simulink model "P702_NI_SoftECU"  (R2019a)
settings: Solver=ode1  StartTime=0.0  StopTime=Inf  FixedStep=0.001  RelTol=1e-3  EnableMultiTasking=on
PreLoadFcn:
  | run '.\VeriStand_BlockSet\NIVeriStandAddPaths.m'
undefined symbols (not defined in the file or in its folder): magnitude
libraries: simulink x83, simulink_extras x1
(part 2 of 76)

== system P702_NI_SoftECU/Input/GWM-SCCM//PDB//RCM//GSM ==
  Bus Creator : BusCreator  Inputs=5
  GMW_Extra_Disable : S-Function  Priority=1  FunctionName=NIVeriStandIO  Parameters=width dtype portnum stime stype btype  SFunctionDeploymentMode=off  EnableBusSupport=off  mask(NI VeriStand Inport){portnum=1, width=-1, stime=-1, dtype=auto, stype=auto, btype=1}
      mask prompts: portnum "Port number:"; width "Port dimensions (-1 for dynamically sized):"; stime "Sample time (-1 for inherited):"; dtype "Data type:"; stype "Signal type:"; btype "Block type:"
      mask help: Use this inport on any level of nested subsystems to allow NI VeriStand software to map signals to it.
      mask init:
      | NIVeriStandIO_init;
      settings: CopyFcn=NIVeriStand_MDL_functions('', 'IO_copy');  DeleteFcn=NIVeriStand_MDL_functions('', 'IO_delete');  MoveFcn=set_param(gcb, 'Mask', 'on');
      mask Callback portnum: NIVeriStand_MDL_functions('', 'IO_setportnum');
      mask TypeOptions dtype: auto | double | single | int8 | uint8 | int16 | uint16 | int32 | uint32 | boolean
      mask Callback dtype: NIVeriStand_MDL_functions('', 'IO_booleansignal');
      mask TypeOptions stype: auto | real | complex
      mask Display:
      | patch([-x x], [-y y], [.90980 .81960 .32156]);
      | plot([xrad -x x xrad], [yrad -y y yrad]);
      | fprintf('NI In%d', portnum);
  GSM : Subsystem  TreatAsAtomicUnit=on
  GSM_Disable : S-Function  Priority=2  FunctionName=NIVeriStandIO  Parameters=width dtype portnum stime stype btype  SFunctionDeploymentMode=off  EnableBusSupport=off  mask(NI VeriStand Inport){portnum=2, width=-1, stime=-1, dtype=auto, stype=auto, btype=1}
      mask prompts: portnum "Port number:"; width "Port dimensions (-1 for dynamically sized):"; stime "Sample time (-1 for inherited):"; dtype "Data type:"; stype "Signal type:"; btype "Block type:"
      mask help: Use this inport on any level of nested subsystems to allow NI VeriStand software to map signals to it.
      mask init:
      | NIVeriStandIO_init;
      settings: CopyFcn=NIVeriStand_MDL_functions('', 'IO_copy');  DeleteFcn=NIVeriStand_MDL_functions('', 'IO_delete');  MoveFcn=set_param(gcb, 'Mask', 'on');
      mask Callback portnum: NIVeriStand_MDL_functions('', 'IO_setportnum');
      mask TypeOptions dtype: auto | double | single | int8 | uint8 | int16 | uint16 | int32 | uint32 | boolean
      mask Callback dtype: NIVeriStand_MDL_functions('', 'IO_booleansignal');
      mask TypeOptions stype: auto | real | complex
      mask Display:
      | patch([-x x], [-y y], [.90980 .81960 .32156]);
      | plot([xrad -x x xrad], [yrad -y y yrad]);
      | fprintf('NI In%d', portnum);
  Other_GWMTx : Subsystem  TreatAsAtomicUnit=on
  RCM : Subsystem  TreatAsAtomicUnit=on
  RCM_Disable : S-Function  Priority=3  FunctionName=NIVeriStandIO  Parameters=width dtype portnum stime stype btype  SFunctionDeploymentMode=off  EnableBusSupport=off  mask(NI VeriStand Inport){portnum=3, width=-1, stime=-1, dtype=auto, stype=auto, btype=1}
      mask prompts: portnum "Port number:"; width "Port dimensions (-1 for dynamically sized):"; stime "Sample time (-1 for inherited):"; dtype "Data type:"; stype "Signal type:"; btype "Block type:"
      mask help: Use this inport on any level of nested subsystems to allow NI VeriStand software to map signals to it.
      mask init:
      | NIVeriStandIO_init;
      settings: CopyFcn=NIVeriStand_MDL_functions('', 'IO_copy');  DeleteFcn=NIVeriStand_MDL_functions('', 'IO_delete');  MoveFcn=set_param(gcb, 'Mask', 'on');
      mask Callback portnum: NIVeriStand_MDL_functions('', 'IO_setportnum');
      mask TypeOptions dtype: auto | double | single | int8 | uint8 | int16 | uint16 | int32 | uint32 | boolean
      mask Callback dtype: NIVeriStand_MDL_functions('', 'IO_booleansignal');
      mask TypeOptions stype: auto | real | complex
      mask Display:
      | patch([-x x], [-y y], [.90980 .81960 .32156]);
      | plot([xrad -x x xrad], [yrad -y y yrad]);
      | fprintf('NI In%d', portnum);
  SCCM : Subsystem  TreatAsAtomicUnit=on
  SCCM_Disable : S-Function  Priority=4  FunctionName=NIVeriStandIO  Parameters=width dtype portnum stime stype btype  SFunctionDeploymentMode=off  EnableBusSupport=off  mask(NI VeriStand Inport){portnum=4, width=-1, stime=-1, dtype=auto, stype=auto, btype=1}
      mask prompts: portnum "Port number:"; width "Port dimensions (-1 for dynamically sized):"; stime "Sample time (-1 for inherited):"; dtype "Data type:"; stype "Signal type:"; btype "Block type:"
      mask help: Use this inport on any level of nested subsystems to allow NI VeriStand software to map signals to it.
      mask init:
      | NIVeriStandIO_init;
      settings: CopyFcn=NIVeriStand_MDL_functions('', 'IO_copy');  DeleteFcn=NIVeriStand_MDL_functions('', 'IO_delete');  MoveFcn=set_param(gcb, 'Mask', 'on');
      mask Callback portnum: NIVeriStand_MDL_functions('', 'IO_setportnum');
      mask TypeOptions dtype: auto | double | single | int8 | uint8 | int16 | uint16 | int32 | uint32 | boolean
      mask Callback dtype: NIVeriStand_MDL_functions('', 'IO_booleansignal');
      mask TypeOptions stype: auto | real | complex
      mask Display:
      | patch([-x x], [-y y], [.90980 .81960 .32156]);
      | plot([xrad -x x xrad], [yrad -y y yrad]);
      | fprintf('NI In%d', portnum);
  Tester/AutoSar : Subsystem  TreatAsAtomicUnit=on
  Tstr/AutoSar_Disable : S-Function  Priority=5  FunctionName=NIVeriStandIO  Parameters=width dtype portnum stime stype btype  SFunctionDeploymentMode=off  EnableBusSupport=off  mask(NI VeriStand Inport){portnum=5, width=-1, stime=-1, dtype=auto, stype=auto, btype=1}
      mask prompts: portnum "Port number:"; width "Port dimensions (-1 for dynamically sized):"; stime "Sample time (-1 for inherited):"; dtype "Data type:"; stype "Signal type:"; btype "Block type:"
      mask help: Use this inport on any level of nested subsystems to allow NI VeriStand software to map signals to it.
      mask init:
      | NIVeriStandIO_init;
      settings: CopyFcn=NIVeriStand_MDL_functions('', 'IO_copy');  DeleteFcn=NIVeriStand_MDL_functions('', 'IO_delete');  MoveFcn=set_param(gcb, 'Mask', 'on');
      mask Callback portnum: NIVeriStand_MDL_functions('', 'IO_setportnum');
      mask TypeOptions dtype: auto | double | single | int8 | uint8 | int16 | uint16 | int32 | uint32 | boolean
      mask Callback dtype: NIVeriStand_MDL_functions('', 'IO_booleansignal');
      mask TypeOptions stype: auto | real | complex
      mask Display:
      | patch([-x x], [-y y], [.90980 .81960 .32156]);
      | plot([xrad -x x xrad], [yrad -y y yrad]);
      | fprintf('NI In%d', portnum);
  GWM_FD1 : Outport
  wires:
  Bus Creator/1 -> GWM_FD1/1
  Other_GWMTx/1(Other_GWMTx) -> Bus Creator/1  "Other_GWMTx"
  RCM/1(RCM_Signals) -> Bus Creator/2  "RCM"
  SCCM/1(SCCM_Signals) -> Bus Creator/3  "SCCM"
  GSM/1(GSM_Signals) -> Bus Creator/4  "GSM"
  GMW_Extra_Disable/1 -> Other_GWMTx/Enable
  RCM_Disable/1 -> RCM/Enable
  SCCM_Disable/1 -> SCCM/Enable
  GSM_Disable/1 -> GSM/Enable
  Tstr/AutoSar_Disable/1 -> Tester/AutoSar/Enable
  Tester/AutoSar/1(Tester/AutoSar) -> Bus Creator/5  "Tester/AutoSar"

== system P702_NI_SoftECU/Input/PSCM ==
  Enable : EnablePort
  Bus_Msg : BusCreator  Inputs=6
  EPAS_INFO_0x82 : Subsystem
  Lane_Assist_Data3_FD1_0x3CC : Subsystem
  PSCM_AutoSar_NetwrkMgmt_0x5B5 : Subsystem
  SteeringPinion_Data_0x7E : Subsystem
  TesterPhysicalResPSCM_0x738 : Subsystem
  TrailerAid_Data2_0x417 : Subsystem
  PSCM : Outport
  wires:
  Bus_Msg/1 -> PSCM/1  "PSCM"
  SteeringPinion_Data_0x7E/1(SteeringPinion_Data_0x7E) -> Bus_Msg/1  "SteeringPinion_Data_0x7E"
  EPAS_INFO_0x82/1(EPAS_INFO_0x82) -> Bus_Msg/2  "EPAS_INFO_0x82"
  Lane_Assist_Data3_FD1_0x3CC/1(Lane_Assist_Data3_FD1_0x3CC) -> Bus_Msg/3  "Lane_Assist_Data3_FD1_0x3CC"
  TrailerAid_Data2_0x417/1(TrailerAid_Data2_0x417) -> Bus_Msg/4  "TrailerAid_Data2_0x417"
  PSCM_AutoSar_NetwrkMgmt_0x5B5/1(PSCM_AutoSar_NetwrkMgmt_0x5B5) -> Bus_Msg/5  "PSCM_AutoSar_NetwrkMgmt_0x5B5"
  TesterPhysicalResPSCM_0x738/1(TesterPhysicalResPSCM_0x738) -> Bus_Msg/6  "TesterPhysicalResPSCM_0x738"

== system P702_NI_SoftECU/Input/RealPCM ==
  note: This is the actual speed of the vehcile from PCM
  note: User Input from NI UI
  Bus Creator : BusCreator  Inputs=1
  Bus Creator1 : BusCreator  Inputs=2
  Bus Creator2 : BusCreator  Inputs=3
  Bus Creator3 : BusCreator  Inputs=1
  CcStat_D_Actl : S-Function  Priority=1  FunctionName=NIVeriStandIO  Parameters=width dtype portnum stime stype btype  SFunctionDeploymentMode=off  EnableBusSupport=off  mask(NI VeriStand Inport){portnum=1, width=1, stime=-1, dtype=auto, stype=auto, btype=1}
      mask prompts: portnum "Port number:"; width "Port dimensions (-1 for dynamically sized):"; stime "Sample time (-1 for inherited):"; dtype "Data type:"; stype "Signal type:"; btype "Block type:"
      mask help: Use this inport on any level of nested subsystems to allow NI VeriStand software to map signals to it.
      mask init:
      | NIVeriStandIO_init;
      settings: CopyFcn=NIVeriStand_MDL_functions('', 'IO_copy');  DeleteFcn=NIVeriStand_MDL_functions('', 'IO_delete');  MoveFcn=set_param(gcb, 'Mask', 'on');
      mask Callback portnum: NIVeriStand_MDL_functions('', 'IO_setportnum');
      mask TypeOptions dtype: auto | double | single | int8 | uint8 | int16 | uint16 | int32 | uint32 | boolean
      mask Callback dtype: NIVeriStand_MDL_functions('', 'IO_booleansignal');
      mask TypeOptions stype: auto | real | complex
      mask Display:
      | patch([-x x], [-y y], [.90980 .81960 .32156]);
      | plot([xrad -x x xrad], [yrad -y y yrad]);
      | fprintf('NI In%d', portnum);
  Desired_Speed : S-Function  Priority=4  FunctionName=NIVeriStandIO  Parameters=width dtype portnum stime stype btype  SFunctionDeploymentMode=off  EnableBusSupport=off  mask(NI VeriStand Inport){portnum=4, width=1, stime=-1, dtype=auto, stype=auto, btype=1}
      mask prompts: portnum "Port number:"; width "Port dimensions (-1 for dynamically sized):"; stime "Sample time (-1 for inherited):"; dtype "Data type:"; stype "Signal type:"; btype "Block type:"
      mask help: Use this inport on any level of nested subsystems to allow NI VeriStand software to map signals to it.
      mask init:
      | NIVeriStandIO_init;
      settings: CopyFcn=NIVeriStand_MDL_functions('', 'IO_copy');  DeleteFcn=NIVeriStand_MDL_functions('', 'IO_delete');  MoveFcn=set_param(gcb, 'Mask', 'on');
      mask Callback portnum: NIVeriStand_MDL_functions('', 'IO_setportnum');
      mask TypeOptions dtype: auto | double | single | int8 | uint8 | int16 | uint16 | int32 | uint32 | boolean
      mask Callback dtype: NIVeriStand_MDL_functions('', 'IO_booleansignal');
      mask TypeOptions stype: auto | real | complex
      mask Display:
      | patch([-x x], [-y y], [.90980 .81960 .32156]);
      | plot([xrad -x x xrad], [yrad -y y yrad]);
      | fprintf('NI In%d', portnum);
  PCM_status_user_input : S-Function  Priority=2  FunctionName=NIVeriStandIO  Parameters=width dtype portnum stime stype btype  SFunctionDeploymentMode=off  EnableBusSupport=off  mask(NI VeriStand Inport){portnum=2, width=1, stime=-1, dtype=auto, stype=auto, btype=1}
      mask prompts: portnum "Port number:"; width "Port dimensions (-1 for dynamically sized):"; stime "Sample time (-1 for inherited):"; dtype "Data type:"; stype "Signal type:"; btype "Block type:"
      mask help: Use this inport on any level of nested subsystems to allow NI VeriStand software to map signals to it.
      mask init:
      | NIVeriStandIO_init;
      settings: CopyFcn=NIVeriStand_MDL_functions('', 'IO_copy');  DeleteFcn=NIVeriStand_MDL_functions('', 'IO_delete');  MoveFcn=set_param(gcb, 'Mask', 'on');
      mask Callback portnum: NIVeriStand_MDL_functions('', 'IO_setportnum');
      mask TypeOptions dtype: auto | double | single | int8 | uint8 | int16 | uint16 | int32 | uint32 | boolean
      mask Callback dtype: NIVeriStand_MDL_functions('', 'IO_booleansignal');
      mask TypeOptions stype: auto | real | complex
      mask Display:
      | patch([-x x], [-y y], [.90980 .81960 .32156]);
      | plot([xrad -x x xrad], [yrad -y y yrad]);
      | fprintf('NI In%d', portnum);
  Veh_V_ActlEng : S-Function  Priority=3  FunctionName=NIVeriStandIO  Parameters=width dtype portnum stime stype btype  SFunctionDeploymentMode=off  EnableBusSupport=off  mask(NI VeriStand Inport){portnum=3, width=1, stime=-1, dtype=auto, stype=auto, btype=1}
      mask prompts: portnum "Port number:"; width "Port dimensions (-1 for dynamically sized):"; stime "Sample time (-1 for inherited):"; dtype "Data type:"; stype "Signal type:"; btype "Block type:"
      mask help: Use this inport on any level of nested subsystems to allow NI VeriStand software to map signals to it.
      mask init:
      | NIVeriStandIO_init;
      settings: CopyFcn=NIVeriStand_MDL_functions('', 'IO_copy');  DeleteFcn=NIVeriStand_MDL_functions('', 'IO_delete');  MoveFcn=set_param(gcb, 'Mask', 'on');
      mask Callback portnum: NIVeriStand_MDL_functions('', 'IO_setportnum');
      mask TypeOptions dtype: auto | double | single | int8 | uint8 | int16 | uint16 | int32 | uint32 | boolean
      mask Callback dtype: NIVeriStand_MDL_functions('', 'IO_booleansignal');
      mask TypeOptions stype: auto | real | complex
      mask Display:
      | patch([-x x], [-y y], [.90980 .81960 .32156]);
      | plot([xrad -x x xrad], [yrad -y y yrad]);
      | fprintf('NI In%d', portnum);
  RealPCM : Outport
  wires:
  CcStat_D_Actl/1 -> Bus Creator/1  "CcStat_D_Actl"
  Bus Creator2/1 -> RealPCM/1  "RealPCM"
  Bus Creator/1 -> Bus Creator2/1  "EngBrakeData"
  PCM_status_user_input/1 -> Bus Creator1/1  "PCM_status_user_input"
  Bus Creator1/1 -> Bus Creator2/3  "user_channel"
  Veh_V_ActlEng/1 -> Bus Creator3/1  "Veh_V_ActlEng"
  Desired_Speed/1 -> Bus Creator1/2  "Desired_Speed"
  Bus Creator3/1 -> Bus Creator2/2  "EngVehicleSpThrottle2"

== system P702_NI_SoftECU/Output/ABS_ESC ==
  ABS_ESC_Tx : Inport
  ABS_BrkBst_Data_0x4B0 : Subsystem
  ABS_ESC_Bus : BusSelector  OutputSignals=BrakeSnData_5_0x76,BrakeSnData_3_0x77,BrakeSnData_4_0x7D,DesiredTorqBrk_0x213,WheelData_0x216,BrakeSnData_6_0x414,BrakeSysFeatures_0x415,BrakeSysFeatures_2_0x416,BrakeSysFeatures_3_0x41E,ABS_BrkBst_Data_0x4B0,DesiredTorqBrk_2_0x214
  BrakeSnData_3_0x77 : Subsystem
  BrakeSnData_4_0x7D : Subsystem
  BrakeSnData_5_0x76 : Subsystem
  BrakeSnData_6_0x414 : Subsystem
  BrakeSysFeatures_0x415 : Subsystem
  BrakeSysFeatures_2_0x416 : Subsystem
  BrakeSysFeatures_3_0x41E : Subsystem
  DesiredTorqBrk_0x213 : Subsystem
  DesiredTorqBrk_2_0x214 : Subsystem
  WheelData_0x216 : Subsystem
  wires:
  ABS_ESC_Tx/1 -> ABS_ESC_Bus/1  "ABS_ESC"
  ABS_ESC_Bus/1 -> BrakeSnData_5_0x76/1(BrakeSnData_5_0x76)  "<BrakeSnData_5_0x76>"
  ABS_ESC_Bus/2 -> BrakeSnData_3_0x77/1(BrakeSnData_3_0x77)  "<BrakeSnData_3_0x77>"
  ABS_ESC_Bus/3 -> BrakeSnData_4_0x7D/1(BrakeSnData_4_0x7D)  "<BrakeSnData_4_0x7D>"
  ABS_ESC_Bus/4 -> DesiredTorqBrk_0x213/1(DesiredTorqBrk_0x213)  "<DesiredTorqBrk_0x213>"
  ABS_ESC_Bus/5 -> WheelData_0x216/1(WheelData_0x216)  "<WheelData_0x216>"
  ABS_ESC_Bus/6 -> BrakeSnData_6_0x414/1(BrakeSnData_6_0x414)  "<BrakeSnData_6_0x414>"
  ABS_ESC_Bus/7 -> BrakeSysFeatures_0x415/1(BrakeSysFeatures_0x415)  "<BrakeSysFeatures_0x415>"
  ABS_ESC_Bus/8 -> BrakeSysFeatures_2_0x416/1(BrakeSysFeatures_2_0x416)  "<BrakeSysFeatures_2_0x416>"
  ABS_ESC_Bus/9 -> BrakeSysFeatures_3_0x41E/1(BrakeSysFeatures_3_0x41E)  "<BrakeSysFeatures_3_0x41E>"
  ABS_ESC_Bus/10 -> ABS_BrkBst_Data_0x4B0/1(ABS_BrkBst_Data_0x4B0)  "<ABS_BrkBst_Data_0x4B0>"
  ABS_ESC_Bus/11 -> DesiredTorqBrk_2_0x214/1(DesiredTorqBrk_2_0x214)  "<DesiredTorqBrk_2_0x214>"

== system P702_NI_SoftECU/Output/BCM ==
  BCM_Tx : Inport
  BCM_Bus : BusSelector  OutputSignals=GlobalClock_Data_0x84,BodyInfo_3_0x3B3,Body_Info_4_0x242,BCM_Lamp_Stat_0x3C3,Battery_Mgmt_2_0x42C
  BCM_Lamp_Stat_0x3C3 : Subsystem
  Battery_Mgmt_2 : Subsystem
  BodyInfo_3_0x3B3 : Subsystem
  Body_Info_4_0x242 : Subsystem
  GlobalClock_Data_0x84 : Subsystem
  wires:
  BCM_Tx/1 -> BCM_Bus/1  "BCM"
  BCM_Bus/2 -> BodyInfo_3_0x3B3/1(BodyInfo_3_0x3B3)  "<BodyInfo_3_0x3B3>"
  BCM_Bus/1 -> GlobalClock_Data_0x84/1(GlobalClock_Data_0x84)  "<GlobalClock_Data_0x84>"
  BCM_Bus/3 -> Body_Info_4_0x242/1(Body_Info_4_0x242)  "<Body_Info_4_0x242>"
  BCM_Bus/4 -> BCM_Lamp_Stat_0x3C3/1(BCM_Lamp_Stat_FD1)  "<BCM_Lamp_Stat_0x3C3>"
  BCM_Bus/5 -> Battery_Mgmt_2/1(Battery_Mgmt_2_FD1)  "<Battery_Mgmt_2_0x42C>"

== system P702_NI_SoftECU/Output/DSMC ==
  DSMC : Inport
  Bus_Msg : BusSelector  OutputSignals=CMR_DSMC_AutoSar_NetwrkMgt,DrvStatMonData,TesterPhysicalResCMR_DSMC
  CMR_DSMC_AutoSar_NetwrkMgt : Subsystem  Commented=on
  DrvStatMonData : Subsystem
  TesterPhysicalResCMR_DSMC : Subsystem  Commented=on
  wires:
  Bus_Msg/3 -> TesterPhysicalResCMR_DSMC/1(TesterPhysicalResCMR_DSMC)  "<TesterPhysicalResCMR_DSMC>"
  Bus_Msg/2 -> DrvStatMonData/1(DrvStatMonData)  "<DrvStatMonData>"
  Bus_Msg/1 -> CMR_DSMC_AutoSar_NetwrkMgt/1(CMR_DSMC_AutoSar_NetwrkMgt)  "<CMR_DSMC_AutoSar_NetwrkMgt>"
  DSMC/1 -> Bus_Msg/1

== system P702_NI_SoftECU/Output/ECM_DIESEL PCM PCM_HEV ==
  ECM_DIESEL PCM PCM_HEV_Tx : Inport
  <Engine_Clutch_Data_0x42F> : Subsystem
  ECM_DIESEL PCM PCM_HEV_Bus : BusSelector  OutputSignals=EngBrakeData_0x165,VehicleOperatingModes_0x167,EngineClimateData_0x178,EngineData_7_0x179,TorqueDataEngFlags_0x200,EngVehicleSpThrottle2_0x202,EngVehicleSpThrottle_0x204,PowertrainData_6_0x205,PowertrainData_3_0x43E,Powertrain_Data_5_0x43F,Gear_Shift_by_Wire_3,PowertrainData_10,TransGearData,HEV_Powertrain_Data2,Global_PATS_TargetInfo_0x47,Engine_Clutch_Data_0x42F
  EngBrakeData_0x165 : Subsystem
  EngVehicleSpThrottle2_0x202 : Subsystem
  EngVehicleSpThrottle_0x204 : Subsystem
  EngineClimateData_0x178 : Subsystem
  EngineData_7_0x179 : Subsystem
  Gear_Shift_by_Wire_3 : Subsystem
  Global_PATS_TargetInfo_0x47 : Subsystem
  HEV_Powertrain_Data2 : Subsystem
  PowertrainData_10 : Subsystem
  PowertrainData_3_0x43E : Subsystem
  PowertrainData_6_0x205 : Subsystem
  Powertrain_Data_5_0x43F : Subsystem
  TorqueDataEngFlags_0x200 : Subsystem
  TransGearData : Subsystem
  VehicleOperatingModes_0x167 : Subsystem
  wires:
  ECM_DIESEL PCM PCM_HEV_Tx/1 -> ECM_DIESEL PCM PCM_HEV_Bus/1  "ECM_DIESEL PCM PCM_HEV"
  ECM_DIESEL PCM PCM_HEV_Bus/7 -> EngVehicleSpThrottle_0x204/1(EngVehicleSpThrottle_0x204)  "<EngVehicleSpThrottle_0x204>"
  ECM_DIESEL PCM PCM_HEV_Bus/5 -> TorqueDataEngFlags_0x200/1(TorqueDataEngFlags_0x200)  "<TorqueDataEngFlags_0x200>"
  ECM_DIESEL PCM PCM_HEV_Bus/6 -> EngVehicleSpThrottle2_0x202/1(EngVehicleSpThrottle2_0x202)  "<EngVehicleSpThrottle2_0x202>"
  ECM_DIESEL PCM PCM_HEV_Bus/4 -> EngineData_7_0x179/1(EngineData_7_0x179)  "<EngineData_7_0x179>"
  ECM_DIESEL PCM PCM_HEV_Bus/3 -> EngineClimateData_0x178/1(EngineClimateData_0x178)  "<EngineClimateData_0x178>"
  ECM_DIESEL PCM PCM_HEV_Bus/2 -> VehicleOperatingModes_0x167/1(VehicleOperatingModes_0x167)  "<VehicleOperatingModes_0x167>"
  ECM_DIESEL PCM PCM_HEV_Bus/1 -> EngBrakeData_0x165/1(EngBrakeData_0x165)  "<EngBrakeData_0x165>"
  ECM_DIESEL PCM PCM_HEV_Bus/14 -> HEV_Powertrain_Data2/1(<HEV_Powertrain_Data2>)  "<HEV_Powertrain_Data2>"
  ECM_DIESEL PCM PCM_HEV_Bus/8 -> PowertrainData_6_0x205/1(PowertrainData_6_0x205)  "<PowertrainData_6_0x205>"
  ECM_DIESEL PCM PCM_HEV_Bus/9 -> PowertrainData_3_0x43E/1(PowertrainData_3_0x43E)  "<PowertrainData_3_0x43E>"
  ECM_DIESEL PCM PCM_HEV_Bus/10 -> Powertrain_Data_5_0x43F/1(Powertrain_Data_5_0x43F)  "<Powertrain_Data_5_0x43F>"
  ECM_DIESEL PCM PCM_HEV_Bus/11 -> Gear_Shift_by_Wire_3/1(<Gear_Shift_by_Wire_3>)  "<Gear_Shift_by_Wire_3>"
  ECM_DIESEL PCM PCM_HEV_Bus/12 -> PowertrainData_10/1(<PowertrainData_10>)  "<PowertrainData_10>"
  ECM_DIESEL PCM PCM_HEV_Bus/13 -> TransGearData/1(<TransGearData>)  "<TransGearData>"
  ECM_DIESEL PCM PCM_HEV_Bus/15 -> Global_PATS_TargetInfo_0x47/1(Global_PATS_TargetInfo_0x47)  "<Global_PATS_TargetInfo_0x47>"
  ECM_DIESEL PCM PCM_HEV_Bus/16 -> <Engine_Clutch_Data_0x42F>/1(Engine_Clutch_Data)  "<Engine_Clutch_Data_0x42F>"

== system P702_NI_SoftECU/Output/GWM ==
  GWM_Tx : Inport
  GSM : Subsystem
  GWM_Bus : BusSelector  OutputSignals=RCM,SCCM,GSM,Tester/AutoSar,Other_GWMTx
  Other_GWMTx : Subsystem
  RCM : Subsystem
  SCCM : Subsystem
  Tester/AutoSar : Subsystem
  wires:
  GWM_Tx/1 -> GWM_Bus/1  "GWM_Tx"
  GWM_Bus/1 -> RCM/1(RCM_Tx_1)  "<RCM>"
  GWM_Bus/2 -> SCCM/1(SCCM)  "<SCCM>"
  GWM_Bus/3 -> GSM/1(GSM)  "<GSM>"
  GWM_Bus/4 -> Tester/AutoSar/1(Tester/AutoSar)  "<Tester/AutoSar>"
  GWM_Bus/5 -> Other_GWMTx/1(Other_GWMTx)  "<Other_GWMTx>"

== system P702_NI_SoftECU/Output/PCAN_ADAS ==
  note: 7 dimensions:
      | 1: CAN_DET_RANGE
      | 2: CAN_DET_RANGE_RATE
      | 3: CAN_DET_AZIMUTH
      | 4: CAN_DET_ELEVATION
      | 5:CAN_DET_SUPE_RES_TARGET
      | 6: CAN_DET_AMPLITUDE
      | 7: CAN_DET_VALID_LEVEL
      | Mingqi & Serene18
  In1 : Inport
  MRR_Detection_001 : Subsystem
  MRR_Detection_002 : Subsystem
  MRR_Detection_003 : Subsystem
  SRR_FL_Detection_001 : Subsystem
  SRR_FL_Detection_002 : Subsystem
  SRR_FL_Detection_003 : Subsystem
  SRR_FR_Detection_001 : Subsystem
  SRR_FR_Detection_002 : Subsystem
  SRR_FR_Detection_003 : Subsystem
  SRR_RL_Detection_001 : Subsystem
  SRR_RL_Detection_002 : Subsystem
  SRR_RL_Detection_003 : Subsystem
  SRR_RR_Detection_001 : Subsystem
  SRR_RR_Detection_002 : Subsystem
  SRR_RR_Detection_003 : Subsystem
  wires:
  In1/1 -> MRR_Detection_002/1(in), MRR_Detection_001/1(in), SRR_RR_Detection_002/1(in), SRR_RR_Detection_003/1(in), SRR_FR_Detection_001/1(in), SRR_FR_Detection_002/1(in), SRR_FR_Detection_003/1(in), SRR_RL_Detection_001/1(in), SRR_RL_Detection_002/1(in), SRR_RL_Detection_003/1(in), SRR_FL_Detection_001/1(in), SRR_FL_Detection_002/1(in), SRR_FL_Detection_003/1(in), SRR_RR_Detection_001/1(in), MRR_Detection_003/1(in)

== system P702_NI_SoftECU/Output/PSCM ==
  PSCM_Tx : Inport
  EPAS_INFO_0x82 : Subsystem
  Lane_Assist_Data3_FD1_0x3CC : Subsystem
  PSCM_Bus : BusSelector  OutputSignals=EPAS_INFO_0x82,Lane_Assist_Data3_FD1_0x3CC,TrailerAid_Data2_0x417
  TrailerAid_Data2_0x417 : Subsystem
  wires:
  PSCM_Tx/1 -> PSCM_Bus/1  "PSCM"
  PSCM_Bus/1 -> EPAS_INFO_0x82/1(EPAS_INFO_0x82)  "<EPAS_INFO_0x82>"
  PSCM_Bus/2 -> Lane_Assist_Data3_FD1_0x3CC/1(Lane_Assist_Data3_FD1_0x3CC)  "<Lane_Assist_Data3_FD1_0x3CC>"
  PSCM_Bus/3 -> TrailerAid_Data2_0x417/1(TrailerAid_Data2_0x417)  "<TrailerAid_Data2_0x417>"

== system P702_NI_SoftECU/Output/SoftECULogic_NIXNET_CAN_FD1 ==
  In1 : Inport
  ABS_BrkBst_Data : Subsystem
  Accel_Data_FD1 : Subsystem
  BrakeSnData_3 : Subsystem
  BrakeSnData_4 : Subsystem
  BrakeSnData_5 : Subsystem
  BrakeSysFeatures : Subsystem
  BrakeSysFeatures_2 : Subsystem
  Cluster_Info1_FD1 : Subsystem
  Compare To Constant : simulink/Logic and Bit Operations/Compare To Constant  relop=>=  const=4  OutDataTypeStr=boolean
  DesiredTorqBrk : Subsystem
  DrvStatMonData : Subsystem
  ECU_wakeup_Ing_stat : S-Function  Priority=1  FunctionName=NIVeriStandIO  Parameters=width dtype portnum stime stype btype  SFunctionDeploymentMode=off  EnableBusSupport=off  mask(NI VeriStand Inport){portnum=1, width=-1, stime=-1, dtype=auto, stype=auto, btype=1}
      mask prompts: portnum "Port number:"; width "Port dimensions (-1 for dynamically sized):"; stime "Sample time (-1 for inherited):"; dtype "Data type:"; stype "Signal type:"; btype "Block type:"
      mask help: Use this inport on any level of nested subsystems to allow NI VeriStand software to map signals to it.
      mask init:
      | NIVeriStandIO_init;
      settings: CopyFcn=NIVeriStand_MDL_functions('', 'IO_copy');  DeleteFcn=NIVeriStand_MDL_functions('', 'IO_delete');  MoveFcn=set_param(gcb, 'Mask', 'on');
      mask Callback portnum: NIVeriStand_MDL_functions('', 'IO_setportnum');
      mask TypeOptions dtype: auto | double | single | int8 | uint8 | int16 | uint16 | int32 | uint32 | boolean
      mask Callback dtype: NIVeriStand_MDL_functions('', 'IO_booleansignal');
      mask TypeOptions stype: auto | real | complex
      mask Display:
      | patch([-x x], [-y y], [.90980 .81960 .32156]);
      | plot([xrad -x x xrad], [yrad -y y yrad]);
      | fprintf('NI In%d', portnum);
  EngBrakeData : Subsystem
  EngVehicleSpThrottle : Subsystem
  EngVehicleSpThrottle2 : Subsystem
  GGCC_Config_Mgmt_ID_1_FD1 : Subsystem
  PowertrainData_10 : Subsystem
  RCMStatusMessage2_FD1 : Subsystem
  SteeringPinion_Data : Subsystem
  TorqueDataEngFlags : Subsystem
  TransGearData : Subsystem
  VehicleOperatingModes : Subsystem
  WheelData : Subsystem
  WheelSpeed : Subsystem
  Yaw_Data : Subsystem
  sdfsd1adf : Constant
  wires:
  In1/1 -> BrakeSysFeatures_2/1(in), ABS_BrkBst_Data/1(in), DrvStatMonData/1(in), PowertrainData_10/1(in), Yaw_Data/1(in), WheelSpeed/1(in), WheelData/1(in), VehicleOperatingModes/1(in), TransGearData/1(in), TorqueDataEngFlags/1(in), SteeringPinion_Data/1(in), Cluster_Info1_FD1/1(in), RCMStatusMessage2_FD1/1(in), GGCC_Config_Mgmt_ID_1_FD1/1(in), Accel_Data_FD1/1(in), BrakeSnData_5/1(in), BrakeSnData_3/1(in), BrakeSnData_4/1(in), BrakeSysFeatures/1(in), DesiredTorqBrk/1(in), EngBrakeData/1(in), EngVehicleSpThrottle2/1(in), EngVehicleSpThrottle/1(in)
  ECU_wakeup_Ing_stat/1 -> Compare To Constant/1
  Compare To Constant/1 -> Cluster_Info1_FD1/Enable

== system P702_NI_SoftECU/Output/Subsystem ==
  a/b : Subsystem
  c : Subsystem
  d : Subsystem

== system P702_NI_SoftECU/Output/Subsystem1 ==
  in_port : Inport
  CAN_Signal : Subsystem
  To_NI_HIL : Subsystem
  bus_selector : BusSelector  OutputSignals=To_NI_HIL,CAN_Signal
  wires:
  in_port/1 -> bus_selector/1  "Subsystem1"
  bus_selector/1 -> To_NI_HIL/1(in_port)  "<To_NI_HIL>"
  bus_selector/2 -> CAN_Signal/1(in_port)  "<CAN_Signal>"

== system P702_NI_SoftECU/Output/Subsystem2 ==
  CAN_Signal : Subsystem
  To_NI_HIL : Subsystem
  bus_creator : BusCreator  Inputs=2
  out_port : Outport
  wires:
  bus_creator/1 -> out_port/1  "Subsystem2"
  To_NI_HIL/1(out_port) -> bus_creator/1  "To_NI_HIL"
  CAN_Signal/1(out_port) -> bus_creator/2  "CAN_Signal"

== system P702_NI_SoftECU/SoftECU/ABS ==
  In1 : Inport
  CAN : Inport  Port=2
  Logic : Subsystem
  Mapping : Subsystem
  Out1 : Outport
  wires:
  Logic/1(Out1) -> Mapping/1(In1)
  In1/1 -> Logic/1(In1)
  Mapping/1(Out1) -> Out1/1
  CAN/1 -> Logic/2(CAN)

== system P702_NI_SoftECU/SoftECU/APIM ==
  In1 : Inport
  Out1 : Outport
  wires:
  In1/1 -> Out1/1

== system P702_NI_SoftECU/SoftECU/BCM ==
  In1 : Inport
  Logic : Subsystem
  Mapping : Subsystem
  Out1 : Outport
  wires:
  In1/1 -> Logic/1(In1)
  Mapping/1(Out1) -> Out1/1
  Logic/1(Out1) -> Mapping/1(In1)

== system P702_NI_SoftECU/SoftECU/CCM ==
  In1 : Inport
  Out1 : Outport
  wires:
  In1/1 -> Out1/1

== system P702_NI_SoftECU/SoftECU/DSMC ==
  In1 : Inport
  Logic : Subsystem
  Mapping : Subsystem
  Out1 : Outport
  wires:
  In1/1 -> Logic/1(In1)
  Logic/1(Out1) -> Mapping/1(In1)
  Mapping/1(Out1) -> Out1/1

== system P702_NI_SoftECU/SoftECU/ECM ==
  In1 : Inport
  CAN : Inport  Port=2
  Logic : Subsystem
  Mapping : Subsystem
  Out1 : Outport
  wires:
  Logic/1(Out1) -> Mapping/1(In1)
  In1/1 -> Logic/1(In1)
  Mapping/1(Out1) -> Out1/1
  CAN/1 -> Mapping/2(CAN)

== system P702_NI_SoftECU/SoftECU/IPC ==
  In1 : Inport
  Out1 : Outport
  wires:
  In1/1 -> Out1/1

== system P702_NI_SoftECU/SoftECU/IPMA ==
  In1 : Inport
  Out1 : Outport
  wires:
  In1/1 -> Out1/1

== system P702_NI_SoftECU/SoftECU/MRR ==
  In1 : Inport
  Logic : Subsystem
  Mapping : Subsystem
  Out1 : Outport
  wires:
  In1/1 -> Logic/1(In1)
  Mapping/1(Out1) -> Out1/1
  Logic/1(Out1) -> Mapping/1(In1)

== system P702_NI_SoftECU/SoftECU/PCM ==
  In1 : Inport
  CAN : Inport  Port=2
  In2 : Inport  Port=3
  Logic1 : Subsystem
  Mapping : Subsystem
  Out1 : Outport
  wires:
  In1/1 -> Logic1/1(In1)
  Logic1/1(Out1) -> Mapping/1(In1)
  Mapping/1(Out1) -> Out1/1
  CAN/1 -> Logic1/2(CAN)
  In2/1 -> Logic1/3(In2)  "CarSim_TCM"

== system P702_NI_SoftECU/SoftECU/PSCM ==
  In1 : Inport
  Logic : Subsystem
  Mapping : Subsystem
  Out1 : Outport
  wires:
  In1/1 -> Logic/1(In1)
  Mapping/1(Out1) -> Out1/1
  Logic/1(Out1) -> Mapping/1(In1)

== system P702_NI_SoftECU/SoftECU/RCM ==
  In1 : Inport
  Logic : Subsystem
  Mapping : Subsystem
  Out1 : Outport
  wires:
  In1/1 -> Logic/1(In1)
  Mapping/1(Out1) -> Out1/1
  Logic/1(Out1) -> Mapping/1(In1)

== system P702_NI_SoftECU/SoftECU/SCCM ==
  In1 : Inport
  Logic : Subsystem
  Mapping : Subsystem
  Out1 : Outport
  wires:
  Logic/1(Out1) -> Mapping/1(In1)
  In1/1 -> Logic/1(In1)
  Mapping/1(Out1) -> Out1/1

== system P702_NI_SoftECU/SoftECU/SRR_L ==
  In1 : Inport
  Bus Creator : BusCreator  Inputs=2
  Carsim_L : Subsystem
  FrontLeft_SOD : Subsystem
  RearLeft_SOD : Subsystem
  SensorPosition_FL : Subsystem
  SensorPosition_RL : Subsystem
  Out : Outport
  wires:
  RearLeft_SOD/1(RL_SOD) -> Bus Creator/1  "RL_SOD"
  FrontLeft_SOD/1(FL_SOD) -> Bus Creator/2  "FL_SOD"
  Bus Creator/1 -> Out/1
  In1/1 -> FrontLeft_SOD/1(In1), RearLeft_SOD/1(In1)
  SensorPosition_RL/1(SensorPosition) -> RearLeft_SOD/2(Sensor_pos)
  Carsim_L/1(CSP) -> FrontLeft_SOD/3(CSP), RearLeft_SOD/3(CSP)
  SensorPosition_FL/1(SensorPosition) -> FrontLeft_SOD/2(Sensor_pos)

== system P702_NI_SoftECU/SoftECU/SRR_R ==
  In1 : Inport
  Bus Creator : BusCreator  Inputs=2
  Carsim_R : Subsystem
  FrontRight_SOD : Subsystem
  RearRight_SOD : Subsystem
  SensorPosition_FR : Subsystem
  SensorPosition_RR : Subsystem
  Out : Outport
  wires:
  Carsim_R/1(CSP) -> FrontRight_SOD/3(CSP), RearRight_SOD/3(CSP)
  SensorPosition_RR/1(SensorPosition) -> RearRight_SOD/2(Sensor_pos)
  SensorPosition_FR/1(SensorPosition) -> FrontRight_SOD/2(Sensor_pos)
  In1/1 -> FrontRight_SOD/1(In1), RearRight_SOD/1(In1)
  RearRight_SOD/1(RR_SOD) -> Bus Creator/1  "RR_SOD"
  FrontRight_SOD/1(FR_SOD) -> Bus Creator/2  "FR_SOD"
  Bus Creator/1 -> Out/1

== system P702_NI_SoftECU/SoftECU/TCM ==
  In1 : Inport
  Logic : Subsystem
  Mapping : Subsystem
  Out1 : Outport
  wires:
  Logic/1(Out1) -> Mapping/1(In1)
  In1/1 -> Logic/1(In1)
  Mapping/1(Out1) -> Out1/1

== system P702_NI_SoftECU/Input/ABS_ESC/ABS_AutoSar_NetworkMgt_0x596 ==
  ABS_AutoSarNMControl : Constant  Commented=on  Value=0
  ABS_AutoSarNMNodeId : Constant  Commented=on  Value=150
  ABS_AutoSarNMReserved{1..4} (4 alike) : Constant  Commented=on  Value=255
  ABS_GWNMProxy : Constant  Commented=on  Value=255
  ABS_GWOnBoardTester : Constant  Commented=on  Value=255
  Bus_Sig : BusCreator  Inputs=8
  ABS_AutoSar_NetworkMgt_0x596 : Outport
  wires:
  ABS_AutoSarNMReserved4/1 -> Bus_Sig/8  "ABS_AutoSarNMReserved4"
  ABS_AutoSarNMReserved3/1 -> Bus_Sig/7  "ABS_AutoSarNMReserved3"
  ABS_GWNMProxy/1 -> Bus_Sig/6  "ABS_GWNMProxy"
  ABS_GWOnBoardTester/1 -> Bus_Sig/5  "ABS_GWOnBoardTester"
  ABS_AutoSarNMReserved2/1 -> Bus_Sig/4  "ABS_AutoSarNMReserved2"
  ABS_AutoSarNMReserved1/1 -> Bus_Sig/3  "ABS_AutoSarNMReserved1"
  ABS_AutoSarNMControl/1 -> Bus_Sig/2  "ABS_AutoSarNMControl"
  ABS_AutoSarNMNodeId/1 -> Bus_Sig/1  "ABS_AutoSarNMNodeId"
  Bus_Sig/1 -> ABS_AutoSar_NetworkMgt_0x596/1  "ABS_AutoSar_NetworkMgt_0x596"

== system P702_NI_SoftECU/Input/ABS_ESC/ABS_BrkBst_Data_0x4B0 ==
  BrkAutoHold_D_Stat_In : S-Function  Priority=1  FunctionName=NIVeriStandIO  Parameters=width dtype portnum stime stype btype  SFunctionDeploymentMode=off  EnableBusSupport=off  mask(NI VeriStand Inport){portnum=1, width=-1, stime=-1, dtype=auto, stype=auto, btype=1}
      mask prompts: portnum "Port number:"; width "Port dimensions (-1 for dynamically sized):"; stime "Sample time (-1 for inherited):"; dtype "Data type:"; stype "Signal type:"; btype "Block type:"
      mask help: Use this inport on any level of nested subsystems to allow NI VeriStand software to map signals to it.
      mask init:
      | NIVeriStandIO_init;
      settings: CopyFcn=NIVeriStand_MDL_functions('', 'IO_copy');  DeleteFcn=NIVeriStand_MDL_functions('', 'IO_delete');  MoveFcn=set_param(gcb, 'Mask', 'on');
      mask Callback portnum: NIVeriStand_MDL_functions('', 'IO_setportnum');
      mask TypeOptions dtype: auto | double | single | int8 | uint8 | int16 | uint16 | int32 | uint32 | boolean
      mask Callback dtype: NIVeriStand_MDL_functions('', 'IO_booleansignal');
      mask TypeOptions stype: auto | real | complex
      mask Display:
      | patch([-x x], [-y y], [.90980 .81960 .32156]);
      | plot([xrad -x x xrad], [yrad -y y yrad]);
      | fprintf('NI In%d', portnum);
  BrkBstrVac_P_Actl_In : S-Function  Priority=2  FunctionName=NIVeriStandIO  Parameters=width dtype portnum stime stype btype  SFunctionDeploymentMode=off  EnableBusSupport=off  mask(NI VeriStand Inport){portnum=2, width=-1, stime=-1, dtype=auto, stype=auto, btype=1}
      mask prompts: portnum "Port number:"; width "Port dimensions (-1 for dynamically sized):"; stime "Sample time (-1 for inherited):"; dtype "Data type:"; stype "Signal type:"; btype "Block type:"
      mask help: Use this inport on any level of nested subsystems to allow NI VeriStand software to map signals to it.
      mask init:
      | NIVeriStandIO_init;
      settings: CopyFcn=NIVeriStand_MDL_functions('', 'IO_copy');  DeleteFcn=NIVeriStand_MDL_functions('', 'IO_delete');  MoveFcn=set_param(gcb, 'Mask', 'on');
      mask Callback portnum: NIVeriStand_MDL_functions('', 'IO_setportnum');
      mask TypeOptions dtype: auto | double | single | int8 | uint8 | int16 | uint16 | int32 | uint32 | boolean
      mask Callback dtype: NIVeriStand_MDL_functions('', 'IO_booleansignal');
      mask TypeOptions stype: auto | real | complex
      mask Display:
      | patch([-x x], [-y y], [.90980 .81960 .32156]);
      | plot([xrad -x x xrad], [yrad -y y yrad]);
      | fprintf('NI In%d', portnum);
  BrkTotTqRqDrv_No_Cnt_In : S-Function  Priority=3  FunctionName=NIVeriStandIO  Parameters=width dtype portnum stime stype btype  SFunctionDeploymentMode=off  EnableBusSupport=off  mask(NI VeriStand Inport){portnum=3, width=-1, stime=-1, dtype=auto, stype=auto, btype=1}
      mask prompts: portnum "Port number:"; width "Port dimensions (-1 for dynamically sized):"; stime "Sample time (-1 for inherited):"; dtype "Data type:"; stype "Signal type:"; btype "Block type:"
      mask help: Use this inport on any level of nested subsystems to allow NI VeriStand software to map signals to it.
      mask init:
      | NIVeriStandIO_init;
      settings: CopyFcn=NIVeriStand_MDL_functions('', 'IO_copy');  DeleteFcn=NIVeriStand_MDL_functions('', 'IO_delete');  MoveFcn=set_param(gcb, 'Mask', 'on');
      mask Callback portnum: NIVeriStand_MDL_functions('', 'IO_setportnum');
      mask TypeOptions dtype: auto | double | single | int8 | uint8 | int16 | uint16 | int32 | uint32 | boolean
      mask Callback dtype: NIVeriStand_MDL_functions('', 'IO_booleansignal');
      mask TypeOptions stype: auto | real | complex
      mask Display:
      | patch([-x x], [-y y], [.90980 .81960 .32156]);
      | plot([xrad -x x xrad], [yrad -y y yrad]);
      | fprintf('NI In%d', portnum);
  BrkTotTqRqDrv_No_Cs_In : S-Function  Priority=4  FunctionName=NIVeriStandIO  Parameters=width dtype portnum stime stype btype  SFunctionDeploymentMode=off  EnableBusSupport=off  mask(NI VeriStand Inport){portnum=4, width=-1, stime=-1, dtype=auto, stype=auto, btype=1}
      mask prompts: portnum "Port number:"; width "Port dimensions (-1 for dynamically sized):"; stime "Sample time (-1 for inherited):"; dtype "Data type:"; stype "Signal type:"; btype "Block type:"
      mask help: Use this inport on any level of nested subsystems to allow NI VeriStand software to map signals to it.
      mask init:
      | NIVeriStandIO_init;
      settings: CopyFcn=NIVeriStand_MDL_functions('', 'IO_copy');  DeleteFcn=NIVeriStand_MDL_functions('', 'IO_delete');  MoveFcn=set_param(gcb, 'Mask', 'on');
      mask Callback portnum: NIVeriStand_MDL_functions('', 'IO_setportnum');
      mask TypeOptions dtype: auto | double | single | int8 | uint8 | int16 | uint16 | int32 | uint32 | boolean
      mask Callback dtype: NIVeriStand_MDL_functions('', 'IO_booleansignal');
      mask TypeOptions stype: auto | real | complex
      mask Display:
      | patch([-x x], [-y y], [.90980 .81960 .32156]);
      | plot([xrad -x x xrad], [yrad -y y yrad]);
      | fprintf('NI In%d', portnum);
  BrkTot_Tq_RqDrv_In : S-Function  Priority=5  FunctionName=NIVeriStandIO  Parameters=width dtype portnum stime stype btype  SFunctionDeploymentMode=off  EnableBusSupport=off  mask(NI VeriStand Inport){portnum=5, width=-1, stime=-1, dtype=auto, stype=auto, btype=1}
      mask prompts: portnum "Port number:"; width "Port dimensions (-1 for dynamically sized):"; stime "Sample time (-1 for inherited):"; dtype "Data type:"; stype "Signal type:"; btype "Block type:"
      mask help: Use this inport on any level of nested subsystems to allow NI VeriStand software to map signals to it.
      mask init:
      | NIVeriStandIO_init;
      settings: CopyFcn=NIVeriStand_MDL_functions('', 'IO_copy');  DeleteFcn=NIVeriStand_MDL_functions('', 'IO_delete');  MoveFcn=set_param(gcb, 'Mask', 'on');
      mask Callback portnum: NIVeriStand_MDL_functions('', 'IO_setportnum');
      mask TypeOptions dtype: auto | double | single | int8 | uint8 | int16 | uint16 | int32 | uint32 | boolean
      mask Callback dtype: NIVeriStand_MDL_functions('', 'IO_booleansignal');
      mask TypeOptions stype: auto | real | complex
      mask Display:
      | patch([-x x], [-y y], [.90980 .81960 .32156]);
      | plot([xrad -x x xrad], [yrad -y y yrad]);
      | fprintf('NI In%d', portnum);
  Bus_Sig : BusCreator  Inputs=8
  HsaStat_D_Dsply : S-Function  Priority=6  FunctionName=NIVeriStandIO  Parameters=width dtype portnum stime stype btype  SFunctionDeploymentMode=off  EnableBusSupport=off  mask(NI VeriStand Inport){portnum=6, width=-1, stime=-1, dtype=auto, stype=auto, btype=1}
      mask prompts: portnum "Port number:"; width "Port dimensions (-1 for dynamically sized):"; stime "Sample time (-1 for inherited):"; dtype "Data type:"; stype "Signal type:"; btype "Block type:"
      mask help: Use this inport on any level of nested subsystems to allow NI VeriStand software to map signals to it.
      mask init:
      | NIVeriStandIO_init;
      settings: CopyFcn=NIVeriStand_MDL_functions('', 'IO_copy');  DeleteFcn=NIVeriStand_MDL_functions('', 'IO_delete');  MoveFcn=set_param(gcb, 'Mask', 'on');
      mask Callback portnum: NIVeriStand_MDL_functions('', 'IO_setportnum');
      mask TypeOptions dtype: auto | double | single | int8 | uint8 | int16 | uint16 | int32 | uint32 | boolean
      mask Callback dtype: NIVeriStand_MDL_functions('', 'IO_booleansignal');
      mask TypeOptions stype: auto | real | complex
      mask Display:
      | patch([-x x], [-y y], [.90980 .81960 .32156]);
      | plot([xrad -x x xrad], [yrad -y y yrad]);
      | fprintf('NI In%d', portnum);
  HsaTrnAout_Tq_Rq : S-Function  Priority=7  FunctionName=NIVeriStandIO  Parameters=width dtype portnum stime stype btype  SFunctionDeploymentMode=off  EnableBusSupport=off  mask(NI VeriStand Inport){portnum=7, width=-1, stime=-1, dtype=auto, stype=auto, btype=1}
      mask prompts: portnum "Port number:"; width "Port dimensions (-1 for dynamically sized):"; stime "Sample time (-1 for inherited):"; dtype "Data type:"; stype "Signal type:"; btype "Block type:"
      mask help: Use this inport on any level of nested subsystems to allow NI VeriStand software to map signals to it.
      mask init:
      | NIVeriStandIO_init;
      settings: CopyFcn=NIVeriStand_MDL_functions('', 'IO_copy');  DeleteFcn=NIVeriStand_MDL_functions('', 'IO_delete');  MoveFcn=set_param(gcb, 'Mask', 'on');
      mask Callback portnum: NIVeriStand_MDL_functions('', 'IO_setportnum');
      mask TypeOptions dtype: auto | double | single | int8 | uint8 | int16 | uint16 | int32 | uint32 | boolean
      mask Callback dtype: NIVeriStand_MDL_functions('', 'IO_booleansignal');
      mask TypeOptions stype: auto | real | complex
      mask Display:
      | patch([-x x], [-y y], [.90980 .81960 .32156]);
      | plot([xrad -x x xrad], [yrad -y y yrad]);
      | fprintf('NI In%d', portnum);
  YawStabilityIndex : S-Function  Priority=8  FunctionName=NIVeriStandIO  Parameters=width dtype portnum stime stype btype  SFunctionDeploymentMode=off  EnableBusSupport=off  mask(NI VeriStand Inport){portnum=8, width=-1, stime=-1, dtype=auto, stype=auto, btype=1}
      mask prompts: portnum "Port number:"; width "Port dimensions (-1 for dynamically sized):"; stime "Sample time (-1 for inherited):"; dtype "Data type:"; stype "Signal type:"; btype "Block type:"
      mask help: Use this inport on any level of nested subsystems to allow NI VeriStand software to map signals to it.
      mask init:
      | NIVeriStandIO_init;
      settings: CopyFcn=NIVeriStand_MDL_functions('', 'IO_copy');  DeleteFcn=NIVeriStand_MDL_functions('', 'IO_delete');  MoveFcn=set_param(gcb, 'Mask', 'on');
      mask Callback portnum: NIVeriStand_MDL_functions('', 'IO_setportnum');
      mask TypeOptions dtype: auto | double | single | int8 | uint8 | int16 | uint16 | int32 | uint32 | boolean
      mask Callback dtype: NIVeriStand_MDL_functions('', 'IO_booleansignal');
      mask TypeOptions stype: auto | real | complex
      mask Display:
      | patch([-x x], [-y y], [.90980 .81960 .32156]);
      | plot([xrad -x x xrad], [yrad -y y yrad]);
      | fprintf('NI In%d', portnum);
  ABS_BrkBst_Data_0x4B0 : Outport
  wires:
  BrkTotTqRqDrv_No_Cs_In/1 -> Bus_Sig/8  "BrkTotTqRqDrv_No_Cs"
  HsaStat_D_Dsply/1 -> Bus_Sig/7  "HsaStat_D_Dsply"
  BrkTot_Tq_RqDrv_In/1 -> Bus_Sig/6  "BrkTot_Tq_RqDrv"
  BrkAutoHold_D_Stat_In/1 -> Bus_Sig/5  "BrkAutoHold_D_Stat"
  BrkTotTqRqDrv_No_Cnt_In/1 -> Bus_Sig/4  "BrkTotTqRqDrv_No_Cnt"
  HsaTrnAout_Tq_Rq/1 -> Bus_Sig/3  "HsaTrnAout_Tq_Rq"
  YawStabilityIndex/1 -> Bus_Sig/2  "YawStabilityIndex"
  BrkBstrVac_P_Actl_In/1 -> Bus_Sig/1  "BrkBstrVac_P_Actl"
  Bus_Sig/1 -> ABS_BrkBst_Data_0x4B0/1  "ABS_BrkBst_Data_0x4B0"

== system P702_NI_SoftECU/Input/ABS_ESC/ABS_Rapid_Data_Response_1_0x6B0 ==
  Bus_Sig : BusCreator  Inputs=1
  UUDTABSResponse1 : Constant  Commented=on  Value=0
  ABS_Rapid_Data_Response_1_0x6B0 : Outport
  wires:
  UUDTABSResponse1/1 -> Bus_Sig/1  "UUDTABSResponse1"
  Bus_Sig/1 -> ABS_Rapid_Data_Response_1_0x6B0/1  "ABS_Rapid_Data_Response_1_0x6B0"

== system P702_NI_SoftECU/Input/ABS_ESC/ABS_Rapid_Data_Response_2_0x6B1 ==
  Bus_Sig : BusCreator  Inputs=1
  UUDTABSResponse2 : Constant  Commented=on  Value=0
  ABS_Rapid_Data_Response_2_0x6B1 : Outport
  wires:
  UUDTABSResponse2/1 -> Bus_Sig/1  "UUDTABSResponse2"
  Bus_Sig/1 -> ABS_Rapid_Data_Response_2_0x6B1/1  "ABS_Rapid_Data_Response_2_0x6B1"

== system P702_NI_SoftECU/Input/ABS_ESC/ActiveFronSteering_Req_0x88 ==
  Bus_Sig : BusCreator  Inputs=3
  SteWhlBrkAnRq_No_Cnt : Constant  Commented=on  Value=0
  SteWhlBrkAnRq_No_Cs : Constant  Commented=on  Value=0
  SteWhlBrkOffst_An_Rq : Constant  Commented=on  Value=1676.5
  ActiveFronSteering_Req_0x88 : Outport
  wires:
  SteWhlBrkAnRq_No_Cnt/1 -> Bus_Sig/3  "SteWhlBrkAnRq_No_Cnt"
  SteWhlBrkAnRq_No_Cs/1 -> Bus_Sig/2  "SteWhlBrkAnRq_No_Cs"
  SteWhlBrkOffst_An_Rq/1 -> Bus_Sig/1  "SteWhlBrkOffst_An_Rq"
  Bus_Sig/1 -> ActiveFronSteering_Req_0x88/1  "ActiveFronSteering_Req_0x88"

== system P702_NI_SoftECU/Input/ABS_ESC/BrakeSnData_3_0x77 ==
  Bus_Sig : BusCreator  Inputs=5
  VehLatComp_A_Actl_In : Constant
  VehLongComp_A_Actl_In : Constant
  VehOverGnd_V_Est_In : Constant
  VehTrvlDir_D_Stat_In : S-Function  Priority=1  FunctionName=NIVeriStandIO  Parameters=width dtype portnum stime stype btype  SFunctionDeploymentMode=off  EnableBusSupport=off  mask(NI VeriStand Inport){portnum=1, width=-1, stime=-1, dtype=auto, stype=auto, btype=1}
      mask prompts: portnum "Port number:"; width "Port dimensions (-1 for dynamically sized):"; stime "Sample time (-1 for inherited):"; dtype "Data type:"; stype "Signal type:"; btype "Block type:"
      mask help: Use this inport on any level of nested subsystems to allow NI VeriStand software to map signals to it.
      mask init:
      | NIVeriStandIO_init;
      settings: CopyFcn=NIVeriStand_MDL_functions('', 'IO_copy');  DeleteFcn=NIVeriStand_MDL_functions('', 'IO_delete');  MoveFcn=set_param(gcb, 'Mask', 'on');
      mask Callback portnum: NIVeriStand_MDL_functions('', 'IO_setportnum');
      mask TypeOptions dtype: auto | double | single | int8 | uint8 | int16 | uint16 | int32 | uint32 | boolean
      mask Callback dtype: NIVeriStand_MDL_functions('', 'IO_booleansignal');
      mask TypeOptions stype: auto | real | complex
      mask Display:
      | patch([-x x], [-y y], [.90980 .81960 .32156]);
      | plot([xrad -x x xrad], [yrad -y y yrad]);
      | fprintf('NI In%d', portnum);
  VehYawComp_W_Actl_In : Constant
  BrakeSnData_3_0x77 : Outport
  wires:
  VehLongComp_A_Actl_In/1 -> Bus_Sig/5  "VehLongComp_A_Actl"
  VehLatComp_A_Actl_In/1 -> Bus_Sig/4  "VehLatComp_A_Actl"
  VehYawComp_W_Actl_In/1 -> Bus_Sig/3  "VehYawComp_W_Actl"
  VehTrvlDir_D_Stat_In/1 -> Bus_Sig/2  "VehTrvlDir_D_Stat"
  VehOverGnd_V_Est_In/1 -> Bus_Sig/1  "VehOverGnd_V_Est"
  Bus_Sig/1 -> BrakeSnData_3_0x77/1  "BrakeSnData_3_0x77"
